simulink model "C2F"  (R2023b)
settings: Solver=VariableStepAuto  StartTime=0.0  StopTime=10.0  RelTol=1e-3
settings Model: Creator=satyamagrawal  LastModifiedBy=satyamagrawal

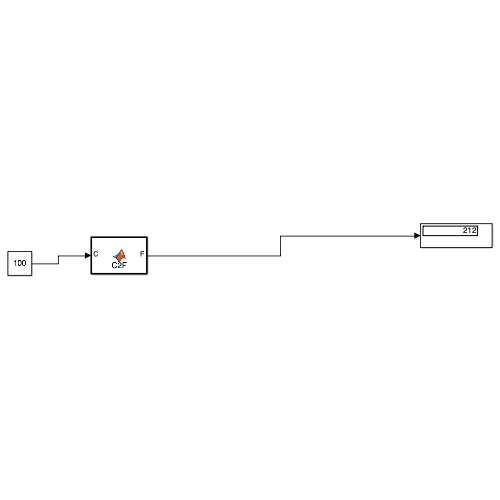
[thumbnail: Simulink's stored preview of the top-level diagram]
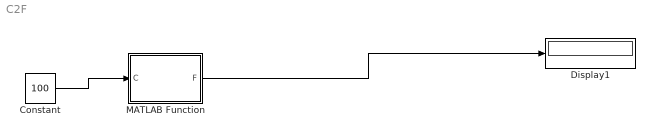
== system C2F ==
  Constant : Constant  Value=100
  Display1 : Display
  MATLAB Function : MATLAB Function  TreatAsAtomicUnit=on
  wires:
  Constant/1 -> MATLAB Function/1(C)
  MATLAB Function/1(F) -> Display1/1

== matlab function C2F/MATLAB Function ==
  data: C input; F output
function F = C2F(C)

F = (C*9/5) + 32;
